simulink model "TestGPS"  (R2016b)
settings: Solver=VariableStepAuto  StartTime=0.0  StopTime=10.0  RelTol=1e-3
model workspace (MAT data in the model file):
  sens = Simulink.Parameter
  sens.Value.rGPS_S_m = [0.3048; 0; 0.0127]
  sens.Value.rGPS_SB_m = [-0.3048; 0; -0.0127]
  sens.Value.errEnable = 1
  sens.Value.posTF_num = 125.663706144
  sens.Value.posTF = [1 125.663706144]
  sens.Value.velTF_num = 125.663706144
  sens.Value.velTF_den = [1 125.663706144]
  sens.Value.timeDelay_s = 0.3
  sens.Value.posScf = [1  0  0; 0  1  0; 0  0  1]
  sens.Value.posBias = [0  0  0; 0  0  0; 0  0  0]
  sens.Value.posSigma = [1e-06; 1e-06; 1]
  sens.Value.posSeed = [6124  21178  9045; 16049  23244  22272; 14601  24729  21466]
  sens.Value.velScf = [1  0  0; 0  1  0; 0  0  1]
  sens.Value.velBias = [0  0  0; 0  0  0; 0  0  0]
  sens.Value.velSigma = [0.1  0.1  0.1; 0.1  0.1  0.1; 0.1  0.1  0.1]
  sens.Value.velSeed = [5329  31448  7334; 3900  11154  24617; 16330  19178  8359]
  sens.Value.timeSample_s = 0.02
  sens.DataType = 'struct'
  sens.Dimensions = [1 1]
libraries: Sensors_Lib x3
settings Model: ParameterArgumentNames=sens  Creator=katiekwiz  LastModifiedBy=katiekwiz

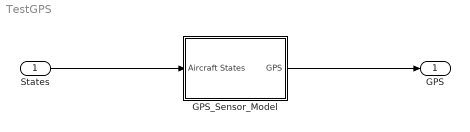
== system TestGPS ==
  States : Inport
  GPS_Sensor_Model : Subsystem  Variant=on  VariantControl=Variant1
  GPS : Outport
  wires:
  States/1 -> GPS_Sensor_Model/1("Aircraft States ")
  GPS_Sensor_Model/1(" GPS") -> GPS/1

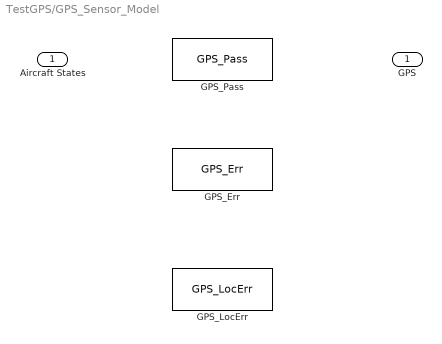
== system TestGPS/GPS_Sensor_Model ==
  "Aircraft States " : Inport
  GPS_Err : Sensors_Lib/GPS Sensor Models/GPS_Err  VariantControl=VarGPS_Err
      settings: AttributesFormatString=Variant: %<VariantControl> : %<Variant>
  GPS_LocErr : Sensors_Lib/GPS Sensor Models/GPS_LocErr  VariantControl=VarGPS_LocErr
      settings: AttributesFormatString=Variant: %<VariantControl> : %<Variant>
  GPS_Pass : Sensors_Lib/GPS Sensor Models/GPS_Pass  VariantControl=VarGPS_Pass
      settings: AttributesFormatString=Variant: %<VariantControl> : %<Variant>
  " GPS" : Outport
